simulink model "carcontrol"  (R2015b)
settings: Solver=VariableStepAuto  StartTime=0.0  StopTime=10.0  RelTol=1e-3
libraries: fuzblock x1
settings Model: Creator=svart  LastModifiedBy=svart

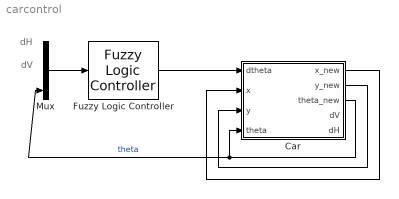
== system carcontrol ==
  note: dH
  note: dV
  Car : MATLAB Function  TreatAsAtomicUnit=on
  Fuzzy Logic Controller : fuzblock/Fuzzy Logic  Controller  fis=flc
  Mux : Mux  Inputs=3
  wires:
  Mux/1 -> Fuzzy Logic Controller/1
  Fuzzy Logic Controller/1 -> Car/1(dtheta)
  Car/2(y_new) -> Car/3(y)
  Car/1(x_new) -> Car/2(x)
  Car/3(theta_new) -> Mux/3, Car/4(theta)  "theta"

== matlab function carcontrol/Car ==
  data: dtheta input; x input; y input; theta input; x_new output; y_new output; theta_new output; dV output; dH output
function [x_new, y_new, theta_new, dV, dH] = carpos(dtheta, x, y, theta)
%#codegen
